simulink subsystem "MagnetoField_magneto"  (R2021a)
settings: Solver=VariableStepAuto  StartTime=0.0  StopTime=10.0  RelTol=1e-3
settings Model: Creator=Laura  LastModifiedBy=Laura

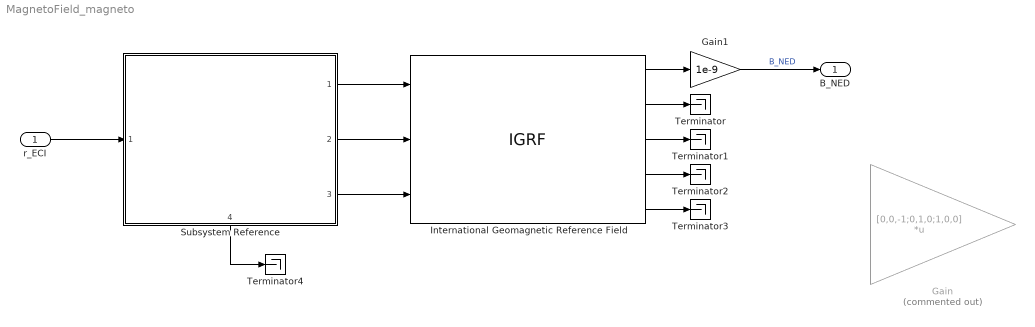
== system MagnetoField_magneto ==
  r_ECI : Inport
  Gain : Gain  Commented=on  Gain=[0,0,-1;0,1,0;1,0,0]  Multiplication=Matrix(K*u)
  Gain1 : Gain  Gain=1e-9
  International Geomagnetic Reference Field : IGRF  time_in=off  month=January  day=1  year=2020  sv_out=off
      settings: AttributesFormatString=%<generation>
  Subsystem Reference : Subsystem  ReferencedSubsystem=ECI2GroundTrack
      settings: PortSchema="{\"entries\":[{\"content\":{\"sides\":[{\"content\":{\"connectorIds\":[\"In1\"]},\"type\":\"ConnectorPlacement.EquallySpacedRectSide\",\"uuid\":\"2c79e801-69ce-474b-a618-0a204c0e6e2c\"},{\"content\":{\"connectorIds\":[\"Out1\",\"Out2\",\"Out3\"],\"side\":\"RIGHT\"},\"type\":\"ConnectorPlacement.EquallySpacedRectSide\",\"uuid\":\"a006009f-cdfc-44f9-9578-b5dfbb39f623\"},{\"content\":{\"connectorIds\":[],\"side\":\"TOP\"},\"type\":\"ConnectorPlacement.EquallySpacedRectSide\",\"uuid\":\"7d10b7e7-37e4-4fd8-9564-aa099ffd2b70\"},{\"content\":{\"connectorIds\":[\"Out4\"],\"side\":\"BOTTOM\"},\"type\":\"ConnectorPlacement.EquallySpacedRectSide\",\"uuid\":\"36e809d8-c229-47c0-82ed-2f1ccf83ce34\"}]},\"type\":\"ConnectorPlacement.EquallySpacedConnector\",\"uuid\":\"0f59f2c7-7320-4754-b018-908c5f0b2a0a\"}],\"packageUris\":[\"http://schema.mathworks.com/mf0/Connector/R2020b\"],\"version\":\"1.0\"}"
  Terminator{,1..4} (5 alike) : Terminator
  B_NED : Outport
  wires:
  International Geomagnetic Reference Field/5 -> Terminator3/1
  Subsystem Reference/1 -> International Geomagnetic Reference Field/1
  International Geomagnetic Reference Field/4 -> Terminator2/1
  International Geomagnetic Reference Field/2 -> Terminator/1
  International Geomagnetic Reference Field/3 -> Terminator1/1
  Subsystem Reference/3 -> International Geomagnetic Reference Field/3
  Subsystem Reference/2 -> International Geomagnetic Reference Field/2
  International Geomagnetic Reference Field/1 -> Gain1/1
  r_ECI/1 -> Subsystem Reference/1
  Gain1/1 -> B_NED/1  "B_NED"
  Subsystem Reference/4 -> Terminator4/1
